simulink library "MuscleLib"  (Simulink 8.3)
settings: Solver=ode45  StartTime=0.0  StopTime=5  RelTol=1e-3
values from neighbouring files (symbols this model uses):
  N = 1000    [modelInit.m]    (also in modelInit_forward.m)
undefined symbols (not defined in the file or in its folder): Newton, Raphson
undefined symbols (not defined in the file): brfactor, l_fore, l_upper
libraries: mblibv1 x6, simulink x1
settings Model: Creator=kbostroem  LastModifiedBy=kbostroem

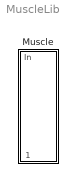
== system MuscleLib ==
  Muscle : Subsystem  mask{PCSA=9.9*brfactor, l_0=0.17, l_tend=sqrt((0.104*l_upper)^2+l_fore^2)-0.17, k1=0.96, k2=0.35, k3=2, lambda=0.22458, lambdaDot=0, Kappa=0.9, Sigma=0.04, delta=0, tau_lambda=0.02, beta_lambda=0.2, lambdaGain=1, lambda_delay=0}
      mask prompts: l_0 "Zero-force length"; l_tend "Tendon length"
      mask init:
      | f_ecc = 1.5;
      | p_fast = 0.6;
      | l_opt = 1.2*l_0;
      | l_max = 4*l_0;
      | f_max = 25*PCSA;
      | lambda_max = 0.5*l_0;
      mask Display:
      | image(imread('icons/muscle.png'));
      | %port_label('lconn', 1, 'C1');
      | %port_label('rconn', 1, 'C2');
      | %port_label('input', 1, 'Force');

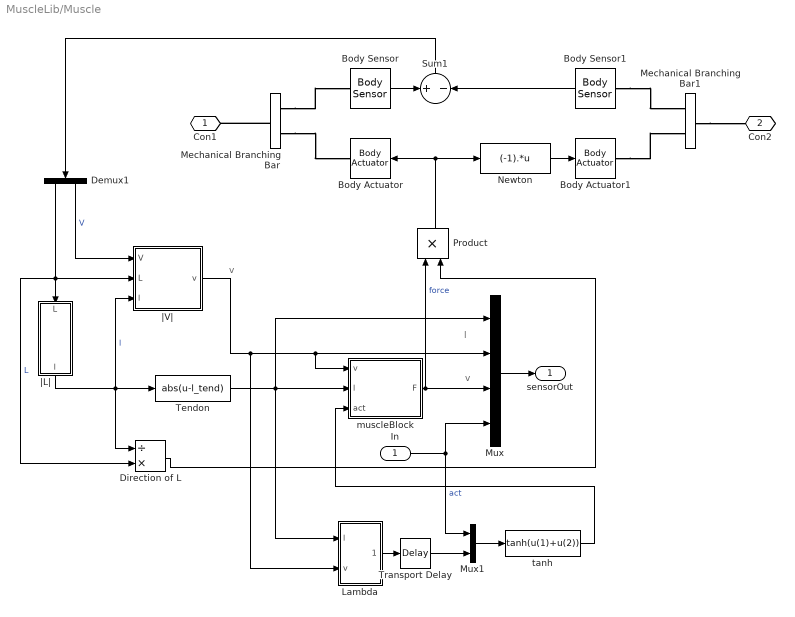
== system MuscleLib/Muscle ==
  note: l
  note: v
  note: v
  In : Inport
  Body Actuator : mblibv1/Sensors &  Actuators/Body Actuator  UpdateFromCAD=off  PhysicalDomain=Mechanical  PortType=blob  ActuationStyle=Force  AngleUnits=deg  ArcVelocityUnits=deg/s  ArcAccelerationUnits=deg/s^2  CoordPositionUnits=m  VelocityUnits=m/s  AccelerationUnits=m/s^2  ForceUnits=N  TorqueUnits=N-m  ActiveIO=off  Width=3  DialogClass=MechanicalActuatorBlock  ReferenceFrame=Absolute (INERTIAL)  Angle=off  CoordPosition=on  Force=on  Torque=off
  Body Actuator1 : mblibv1/Sensors &  Actuators/Body Actuator  UpdateFromCAD=off  PhysicalDomain=Mechanical  PortType=blob  ActuationStyle=Force  AngleUnits=deg  ArcVelocityUnits=deg/s  ArcAccelerationUnits=deg/s^2  CoordPositionUnits=m  VelocityUnits=m/s  AccelerationUnits=m/s^2  ForceUnits=N  TorqueUnits=N*m  ActiveIO=off  Width=3  DialogClass=MechanicalActuatorBlock  ReferenceFrame=Absolute (World)  Angle=off  CoordPosition=on  Force=on  Torque=off
  Body Sensor : mblibv1/Sensors &  Actuators/Body Sensor  UpdateFromCAD=off  PhysicalDomain=Mechanical  PortType=blob  Muxed=on  Pose=off  Angle=on  AngleUnits=deg  ArcVelocity=off  ArcVelocityUnits=deg/s  ArcAcceleration=off  ArcAccelerationUnits=deg/s^2  CoordPosition=on  CoordPositionUnits=m  Velocity=on  VelocityUnits=m/s  Acceleration=off  AccelerationUnits=m/s^2  Quaternion=on  QuaternionDT=off  QuaternionDDT=off  QuaternionUnits=deg  OutputVector=[ 3 3 ]  ActiveIO=off  Width=6  DialogClass=MechanicalSensorBlock  ReferenceFrame=Absolute (World)
  Body Sensor1 : mblibv1/Sensors &  Actuators/Body Sensor  UpdateFromCAD=off  PhysicalDomain=Mechanical  PortType=blob  Muxed=on  Pose=off  Angle=on  AngleUnits=deg  ArcVelocity=off  ArcVelocityUnits=deg/s  ArcAcceleration=off  ArcAccelerationUnits=deg/s^2  CoordPosition=on  CoordPositionUnits=m  Velocity=on  VelocityUnits=m/s  Acceleration=off  AccelerationUnits=m/s^2  Quaternion=on  QuaternionDT=off  QuaternionDDT=off  QuaternionUnits=deg  OutputVector=[ 3 3 ]  ActiveIO=off  Width=6  DialogClass=MechanicalSensorBlock  ReferenceFrame=Absolute (World)
  Demux1 : Demux  Outputs=2
  Direction of L : Product  Inputs=/*
  Lambda : Subsystem  mask{lambda=lambda, lambdaDot=lambdaDot, Kappa=Kappa, Sigma=Sigma, delta=delta, l_opt=l_opt, tau_lambda=tau_lambda, beta_lambda=beta_lambda}
  Mechanical Branching Bar : mblibv1/Utilities/Mechanical Branching Bar  LConnTagsString=_newl0  RConnTagsString=__newr0|SA2  UpdateFromCAD=off  DialogClass=MechanicalBranchingBarBlock  NumSAPorts=2
  Mechanical Branching Bar1 : mblibv1/Utilities/Mechanical Branching Bar  LConnTagsString=_newl0  RConnTagsString=__newr0|SA2  UpdateFromCAD=off  DialogClass=MechanicalBranchingBarBlock  NumSAPorts=2
  Mux : Mux
  Mux1 : Mux  Inputs=2
  Newton : MATLABFcn  MATLABFcn=(-1).*u
  Product : Product  RndMeth=Zero
  Sum1 : Sum  Inputs=+-  SaturateOnIntegerOverflow=on
  Tendon : Fcn  Expr=abs(u-l_tend)
  Transport Delay : TransportDelay  DelayTime=lambda_delay
  muscleBlock : Subsystem  mask{PCSA=PCSA, l_0=l_0, p_fast=p_fast, f_ecc=f_ecc, l_opt=l_opt, l_max=l_max, f_max=f_max, lambda_max=lambda_max, l_tend=l_tend, k1=k1, k2=k2, k3=k3}
      mask init:
      | f_iso = 25*PCSA;
      | v_max = (6+p_fast*10)*l_opt;
      | 
      | a = 0.25*f_iso;
      | b = 0.25*v_max;
      | c = b*(f_iso+a);
      | 
      | a_ecc = f_ecc*f_iso; 
      | b_ecc = (a_ecc-f_iso)*b^2/c; 
      | c_ecc = (a_ecc-f_iso)*b_ecc;
      mask Display:
      | image(imread('icons/muscle.png'));
      | port_label('input', 3, 'Act');
      | port_label('input', 2, 'l');
      | port_label('input', 1, 'v');
      | port_label('output', 1, 'Force');
  tanh : Fcn  Expr=tanh(u(1)+u(2))
  |L| : Subsystem
  |V| : Subsystem
  Con1 : PMIOPort  Port=1  Side=Left
  Con2 : PMIOPort  Port=2  Side=Right
  sensorOut : Outport
  wires:
  muscleBlock/1(F) -> Mux/3, Product/1  "force"
  Newton/1 -> Body Actuator1/1
  Sum1/1 -> Demux1/1
  Body Sensor/1 -> Sum1/1
  Demux1/2 -> |V|/1(V)  "V"
  |V|/1(v) -> Lambda/2(v), Mux/2, muscleBlock/1(v)
  Mux/1 -> sensorOut/1
  Product/1 -> Newton/1, Body Actuator/1
  Body Sensor1/1 -> Sum1/2
  Tendon/1 -> Lambda/1(l), Mux/1, muscleBlock/2(l)
  In/1 -> Mux/4, Mux1/1  "act"
  Direction of L/1 -> Product/2
  Demux1/1 -> Direction of L/2, |L|/1(L), |V|/2(L)  "L"
  |L|/1(l) -> Direction of L/1, Tendon/1, |V|/3(l)  "l"
  Lambda/1(Out1) -> Transport Delay/1
  Mux1/1 -> tanh/1
  Transport Delay/1 -> Mux1/2
  tanh/1 -> muscleBlock/3(act)
  connections:
  Mechanical Branching Bar/LConn1 -- Con1/RConn1
  Body Sensor1/LConn1 -- Mechanical Branching Bar1/RConn1
  Mechanical Branching Bar/RConn1 -- Body Sensor/LConn1
  Mechanical Branching Bar1/LConn1 -- Con2/RConn1
  Mechanical Branching Bar/RConn2 -- Body Actuator/RConn1
  Body Actuator1/RConn1 -- Mechanical Branching Bar1/RConn2

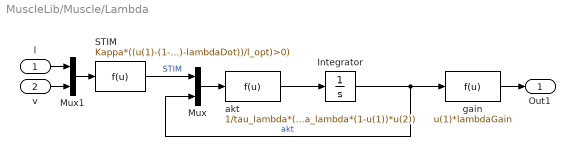
== system MuscleLib/Muscle/Lambda ==
  l : Inport
  v : Inport  Port=2
  Integrator : Integrator
  Mux : Mux  Inputs=2
  Mux1 : Mux  Inputs=2
  STIM : Fcn  Expr=Kappa*((u(1)-(1-delta)*lambda+Sigma*(u(2)-lambdaDot))/l_opt)*(Kappa*((u(1)-(1-delta)*lambda+Sigma*(u(2)-lambdaDot))/l_opt)>0)
  akt : Fcn  Expr=1/tau_lambda*(u(1)*(1-u(2))-beta_lambda*(1-u(1))*u(2))
  gain : Fcn  Expr=u(1)*lambdaGain
  Out1 : Outport
  wires:
  gain/1 -> Out1/1
  v/1 -> Mux1/2
  l/1 -> Mux1/1
  Mux1/1 -> STIM/1
  STIM/1 -> Mux/1  "STIM"
  akt/1 -> Integrator/1
  Mux/1 -> akt/1
  Integrator/1 -> gain/1, Mux/2  "akt"

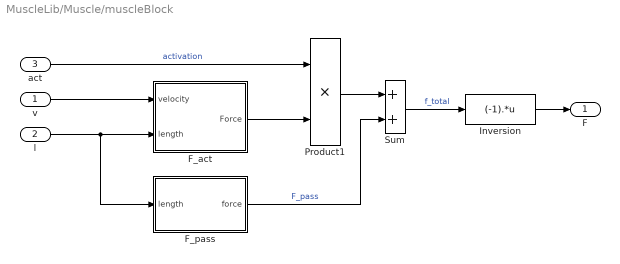
== system MuscleLib/Muscle/muscleBlock ==
  v : Inport
  l : Inport  Port=2
  act : Inport  Port=3
  F_act : Subsystem  Description=active part of the force
  F_pass : Subsystem
  Inversion : MATLABFcn  MATLABFcn=(-1).*u
  Product1 : Product  RndMeth=Zero
  Sum : Sum
  F : Outport
  wires:
  v/1 -> F_act/1(velocity)
  l/1 -> F_pass/1(length), F_act/2(length)
  F_pass/1(force) -> Sum/2  "F_pass"
  Inversion/1 -> F/1
  Sum/1 -> Inversion/1  "f_total"
  Product1/1 -> Sum/1
  F_act/1(Force) -> Product1/2
  act/1 -> Product1/1  "activation"

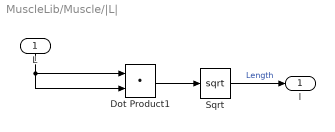
== system MuscleLib/Muscle/|L| ==
  L : Inport
  Dot Product1 : DotProduct  OutDataTypeStr=Inherit: Inherit via internal rule
  Sqrt : Sqrt  AlgorithmType=Newton-Raphson  SaturateOnIntegerOverflow=on
  l : Outport
  wires:
  Dot Product1/1 -> Sqrt/1
  L/1 -> Dot Product1/2, Dot Product1/1
  Sqrt/1 -> l/1  "Length"

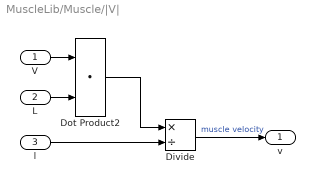
== system MuscleLib/Muscle/|V| ==
  V : Inport
  L : Inport  Port=2
  l : Inport  Port=3
  Divide : Product  Inputs=*/
  Dot Product2 : DotProduct  OutDataTypeStr=Inherit: Inherit via internal rule
  v : Outport
  wires:
  Dot Product2/1 -> Divide/1
  L/1 -> Dot Product2/2
  l/1 -> Divide/2
  V/1 -> Dot Product2/1
  Divide/1 -> v/1  "muscle velocity"

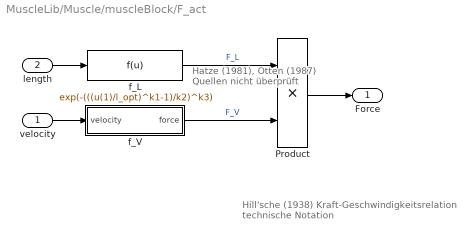
== system MuscleLib/Muscle/muscleBlock/F_act ==
  note: Hill'sche (1938) Kraft-Geschwindigkeitsrelation
      | technische Notation
  note: Hatze (1981), Otten (1987)
      | Quellen nicht überprüft
  velocity : Inport
  length : Inport  Port=2
  Product : Product  RndMeth=Zero
  f_L : Fcn  Expr=exp(-(((u(1)/l_opt)^k1-1)/k2)^k3)
  f_V : Subsystem
  Force : Outport
  wires:
  f_L/1 -> Product/1  "F_L"
  Product/1 -> Force/1
  f_V/1(force) -> Product/2  "F_V"
  length/1 -> f_L/1
  velocity/1 -> f_V/1(velocity)

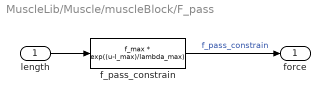
== system MuscleLib/Muscle/muscleBlock/F_pass ==
  length : Inport
  f_pass_constrain : Fcn  Expr=f_max * exp((u-l_max)/lambda_max)
  force : Outport
  wires:
  length/1 -> f_pass_constrain/1
  f_pass_constrain/1 -> force/1  "f_pass_constrain"

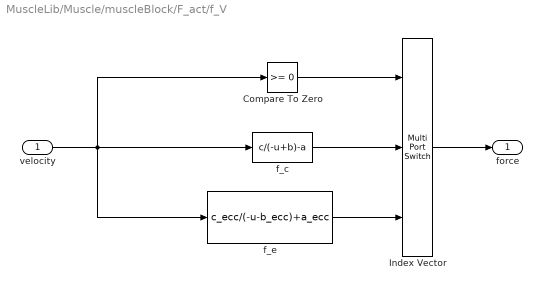
== system MuscleLib/Muscle/muscleBlock/F_act/f_V ==
  velocity : Inport
  Compare To Zero : simulink/Logic and Bit Operations/Compare To Zero  relop=>=  OutDataTypeStr=uint8
  Index Vector : MultiPortSwitch  DataPortOrder=Zero-based contiguous  Inputs=2  zeroidx=on
  f_c : Fcn  Expr=c/(-u+b)-a
  f_e : Fcn  Expr=c_ecc/(-u-b_ecc)+a_ecc
  force : Outport
  wires:
  f_c/1 -> Index Vector/2
  f_e/1 -> Index Vector/3
  Compare To Zero/1 -> Index Vector/1
  velocity/1 -> f_e/1, f_c/1, Compare To Zero/1
  Index Vector/1 -> force/1
